simulink model "yoyo_sim"  (R2015b)
settings: Solver=ode45  StartTime=0.0  StopTime=20  MaxStep=.01  RelTol=1e-3
values from neighbouring files (symbols this model uses):
  d = PARAMS.m*PARAMS.g*PARAMS.r/(PARAMS.I+PARAMS.m*(PARAMS.r^2))    [yoyo_model_simulate.m]
  downA = [0,1;0,-r*epsilon/(I+m*r^2)]    [yoyo_model_simulate.m]
  downB = [0;m*r/(I+m*r^2)]    [yoyo_model_simulate.m]
  downK = [0;m*r*g/(I+m*r^2)]    [yoyo_model_simulate.m]
  newC = [1,0]    [yoyo_model_simulate.m]
  newD = 0    [yoyo_model_simulate.m]
  PARAMS = struct(f1,v1,f2,v2,f3,v3,f4,v4,f5,v5,f6,v6,f7,v7,f8,v8,f9,v9,f10,v10,f11,v11,f12,v12,f13,v13)    [yoyo_model.m]    (also in yoyo_model_simulate.m = struct(f1,v1,f2,v2,f3,v3,f4,v4,f5,v5,f6,v6,f7,v7,f8,v8,f9,v9; yoyo_model_testing_lqi.m)
  upB = [0;-m*r/(I+m*r^2)]    [yoyo_model_simulate.m]
  upK = [0;-m*r*g/(I+m*r^2)]    [yoyo_model_simulate.m]
settings Model: Creator=thomasesch  LastModifiedBy=thomasesch
settings DataIOCC: MaxDataPoints=10000  SaveFormat=Array
settings DebuggingCC: UnderspecifiedInitializationDetection=Classic  MergeDetectMultiDrivingBlocksExec=none  SolverPrmCheckMsg=warning
settings HardwareCC: ProdBitPerPointer=32  ProdLargestAtomicFloat=None  ProdIntDivRoundTo=Undefined  ProdEndianess=Unspecified  ProdWordSize=32  ProdHWDeviceType=32-bit Generic
settings GRTTargetCC: GeneratePreprocessorConditionals=Disable all
settings ConfigComp: CovModelRefEnable=Off

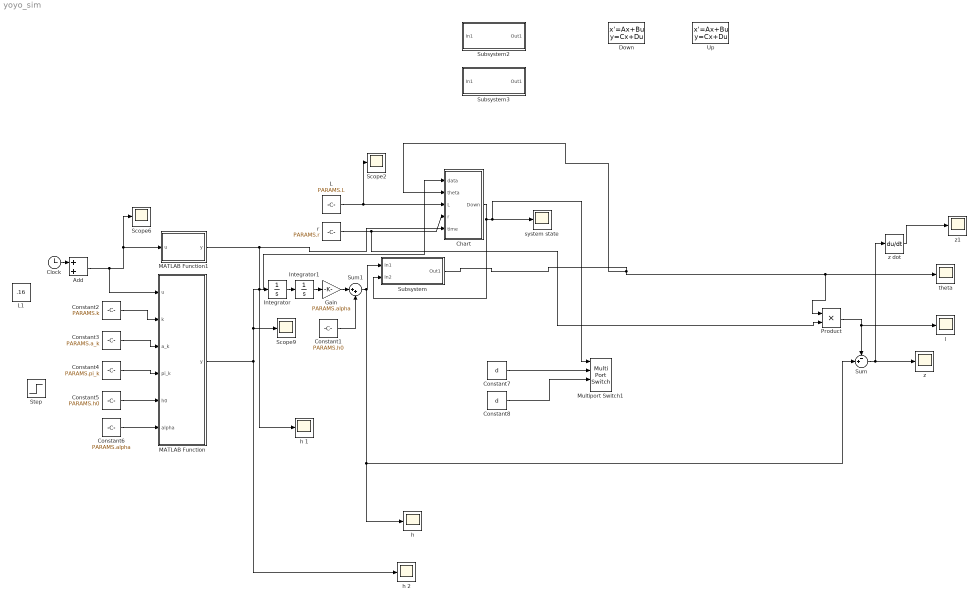
== system yoyo_sim ==
  Add : Sum
  Chart : Stateflow chart  TreatAsAtomicUnit=on
  Clock : Clock
  Constant1 : Constant  Value=PARAMS.h0
  Constant2 : Constant  Value=PARAMS.k
  Constant3 : Constant  Value=PARAMS.a_k
  Constant4 : Constant  Value=PARAMS.pi_k
  Constant5 : Constant  Value=PARAMS.h0
  Constant6 : Constant  Value=PARAMS.alpha
  Constant7 : Constant  Value=d
  Constant8 : Constant  Value=d
  Down : StateSpace  A=downA  B=downB  C=newC  D=0  X0=0
  Gain : Gain  Gain=PARAMS.alpha
  Integrator : Integrator
  Integrator1 : Integrator
  L : Constant  Value=PARAMS.L
  L1 : Constant  Value=.16
  MATLAB Function : MATLAB Function  TreatAsAtomicUnit=on
  MATLAB Function1 : MATLAB Function  TreatAsAtomicUnit=on
  Multiport Switch1 : MultiPortSwitch  DataPortOrder=Zero-based contiguous  Inputs=2  DataPortForDefault=Additional data port
  Product : Product
  Scope2 : Scope
  Scope6 : Scope
  Scope9 : Scope
  Step : Step  SampleTime=0
  Subsystem : Subsystem
  Subsystem2 : Subsystem
  Subsystem3 : Subsystem
  Sum : Sum  Inputs=-+|
  Sum1 : Sum  Inputs=|++
  Up : StateSpace  A=downA  B=upB  C=newC  D=0  X0=0
  "h " : Scope
  h 1 : Scope
  h 2 : Scope
  l : Scope
  r : Constant  Value=PARAMS.r
  system state : Scope
  theta : Scope
  z : Scope
  z dot : Derivative
  z1 : Scope
  wires:
  Integrator/1 -> Integrator1/1
  Integrator1/1 -> Gain/1
  Chart/1(Down) -> Subsystem/2(In2), Multiport Switch1/1, system state/1
  r/1 -> Product/2, Chart/4(r)
  L/1 -> Scope2/1, Chart/3(L)
  Subsystem/1(Out1) -> Product/1, theta/1, Chart/2(theta)
  Constant2/1 -> MATLAB Function/2(k)
  Constant3/1 -> MATLAB Function/3(a_k)
  Constant4/1 -> MATLAB Function/4(pi_k)
  Constant5/1 -> MATLAB Function/5(h0)
  Constant6/1 -> MATLAB Function/6(alpha)
  Product/1 -> l/1, Sum/1
  Sum/1 -> z/1, z dot/1
  Constant7/1 -> Multiport Switch1/2
  Constant8/1 -> Multiport Switch1/3
  z dot/1 -> z1/1
  MATLAB Function1/1(y) -> Chart/5(time), h 1/1
  Clock/1 -> Add/1
  Add/1 -> MATLAB Function/1(u), Scope6/1, MATLAB Function1/1(u)
  MATLAB Function/1(y) -> h 2/1, Chart/1(data), Integrator/1, Scope9/1
  Constant1/1 -> Sum1/2
  Gain/1 -> Sum1/1
  Sum1/1 -> "h "/1, Sum/2, Subsystem/1(In1)

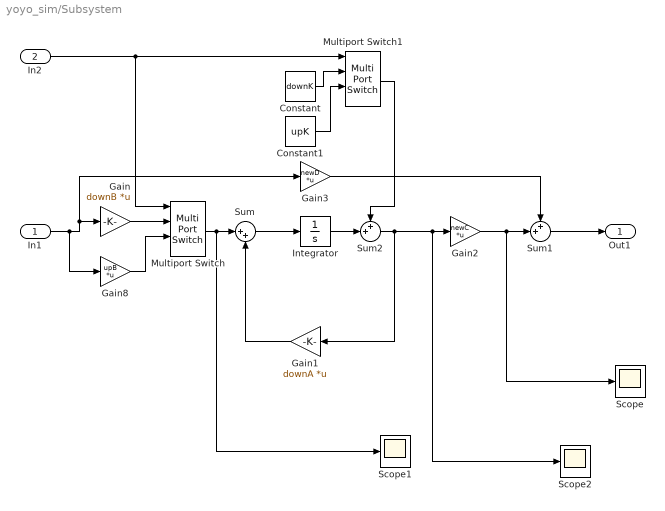
== system yoyo_sim/Subsystem ==
  In1 : Inport
  In2 : Inport  Port=2
  Constant : Constant  Value=downK  VectorParams1D=off
  Constant1 : Constant  Value=upK  VectorParams1D=off
  Gain : Gain  Gain=downB  Multiplication=Matrix(K*u)
  Gain1 : Gain  Gain=downA  Multiplication=Matrix(K*u)
  Gain2 : Gain  Gain=newC  Multiplication=Matrix(K*u)
  Gain3 : Gain  Gain=newD  Multiplication=Matrix(K*u)
  Gain8 : Gain  Gain=upB  Multiplication=Matrix(K*u)
  Integrator : Integrator
  Multiport Switch : MultiPortSwitch  DataPortOrder=Zero-based contiguous  Inputs=2  DataPortForDefault=Additional data port
  Multiport Switch1 : MultiPortSwitch  DataPortOrder=Zero-based contiguous  Inputs=2  DataPortForDefault=Additional data port
  Scope : Scope
  Scope1 : Scope
  Scope2 : Scope
  Sum : Sum  Inputs=|++
  Sum1 : Sum  Inputs=++|
  Sum2 : Sum  Inputs=++|
  Out1 : Outport
  wires:
  In1/1 -> Gain8/1, Gain/1, Gain3/1
  Gain1/1 -> Sum/2
  Sum/1 -> Integrator/1
  Gain3/1 -> Sum1/1
  Gain2/1 -> Scope/1, Sum1/2
  Sum1/1 -> Out1/1
  Integrator/1 -> Sum2/2
  Sum2/1 -> Scope2/1, Gain2/1, Gain1/1
  Gain8/1 -> Multiport Switch/3
  Gain/1 -> Multiport Switch/2
  Multiport Switch/1 -> Scope1/1, Sum/1
  Multiport Switch1/1 -> Sum2/1
  In2/1 -> Multiport Switch/1, Multiport Switch1/1
  Constant1/1 -> Multiport Switch1/3
  Constant/1 -> Multiport Switch1/2

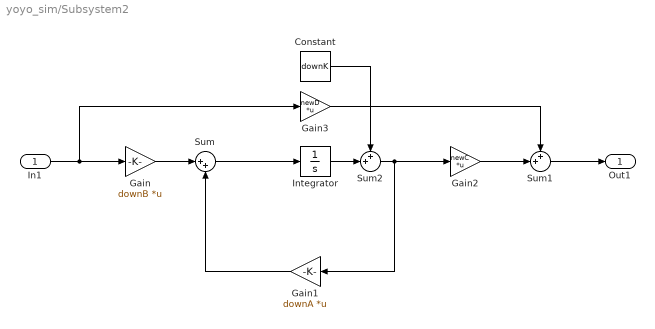
== system yoyo_sim/Subsystem2 ==
  In1 : Inport
  Constant : Constant  Value=downK  VectorParams1D=off
  Gain : Gain  Gain=downB  Multiplication=Matrix(K*u)
  Gain1 : Gain  Gain=downA  Multiplication=Matrix(K*u)
  Gain2 : Gain  Gain=newC  Multiplication=Matrix(K*u)
  Gain3 : Gain  Gain=newD  Multiplication=Matrix(K*u)
  Integrator : Integrator
  Sum : Sum  Inputs=|++
  Sum1 : Sum  Inputs=++|
  Sum2 : Sum  Inputs=++|
  Out1 : Outport
  wires:
  In1/1 -> Gain3/1, Gain/1
  Gain1/1 -> Sum/2
  Gain/1 -> Sum/1
  Sum/1 -> Integrator/1
  Gain3/1 -> Sum1/1
  Gain2/1 -> Sum1/2
  Sum1/1 -> Out1/1
  Integrator/1 -> Sum2/2
  Constant/1 -> Sum2/1
  Sum2/1 -> Gain2/1, Gain1/1

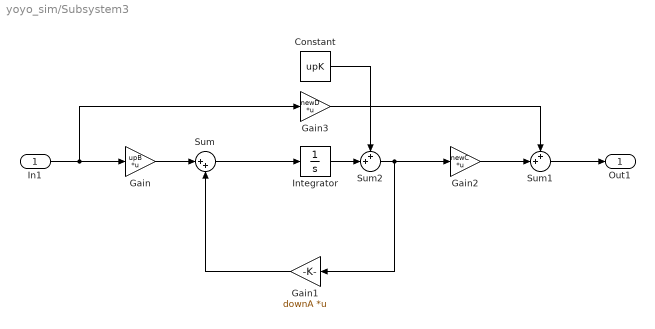
== system yoyo_sim/Subsystem3 ==
  In1 : Inport
  Constant : Constant  Value=upK  VectorParams1D=off
  Gain : Gain  Gain=upB  Multiplication=Matrix(K*u)
  Gain1 : Gain  Gain=downA  Multiplication=Matrix(K*u)
  Gain2 : Gain  Gain=newC  Multiplication=Matrix(K*u)
  Gain3 : Gain  Gain=newD  Multiplication=Matrix(K*u)
  Integrator : Integrator
  Sum : Sum  Inputs=|++
  Sum1 : Sum  Inputs=++|
  Sum2 : Sum  Inputs=++|
  Out1 : Outport
  wires:
  In1/1 -> Gain3/1, Gain/1
  Gain1/1 -> Sum/2
  Gain/1 -> Sum/1
  Sum/1 -> Integrator/1
  Gain3/1 -> Sum1/1
  Gain2/1 -> Sum1/2
  Sum1/1 -> Out1/1
  Integrator/1 -> Sum2/2
  Constant/1 -> Sum2/1
  Sum2/1 -> Gain2/1, Gain1/1

== stateflow chart yoyo_sim/Chart ==
  state Up
    during: Down =1;
  state goingd
    during: Down = 0;
  (default) -> goingd
  goingd -> Up : [r*theta >= L]
  Up -> goingd : [time <=.01]
  data: data input; theta input; L input; r input; Down output double; time input

== matlab function yoyo_sim/MATLAB Function ==
  data: u input; y output; k input; a_k input; pi_k input; h0 input; alpha input
function y = fcn(u,k,a_k,pi_k,h0,alpha)
%#codegen


hot = 0;
for k = 1:k
    hot = hot + a_k(k)*sin(pi_k(k)*u);
end
%hot = h0 + alpha*hot;


y = hot;

== matlab function yoyo_sim/MATLAB Function1 ==
  data: u input; y output
function y = fcn(u)
%#codegen
t = mod((u),1.9);
y = t;
